simulink model "css"  (R2016a)
settings: Solver=ode45  StartTime=0.0  StopTime=inf  RelTol=1e-3
libraries: commfilt2 x3, commrflib2 x2, commrandsrc2 x2, commchan3 x1, commdigbbndam3 x1, dspspect3 x1
settings Model: Creator=NhatPham  LastModifiedBy=Nhat Pham
settings DataIOCC: LimitDataPoints=on  SaveFormat=Array
settings DebuggingCC: SolverPrmCheckMsg=warning
settings HardwareCC: ProdBitPerPointer=32  ProdLargestAtomicFloat=None  ProdIntDivRoundTo=Undefined  ProdEndianess=Unspecified  ProdWordSize=32  ProdHWDeviceType=32-bit Generic
settings ModelReferenceCC: PropagateSignalLabelsOutOfModel=off
settings ConfigComp: CovModelRefEnable=Off  CovSFcnEnable=off

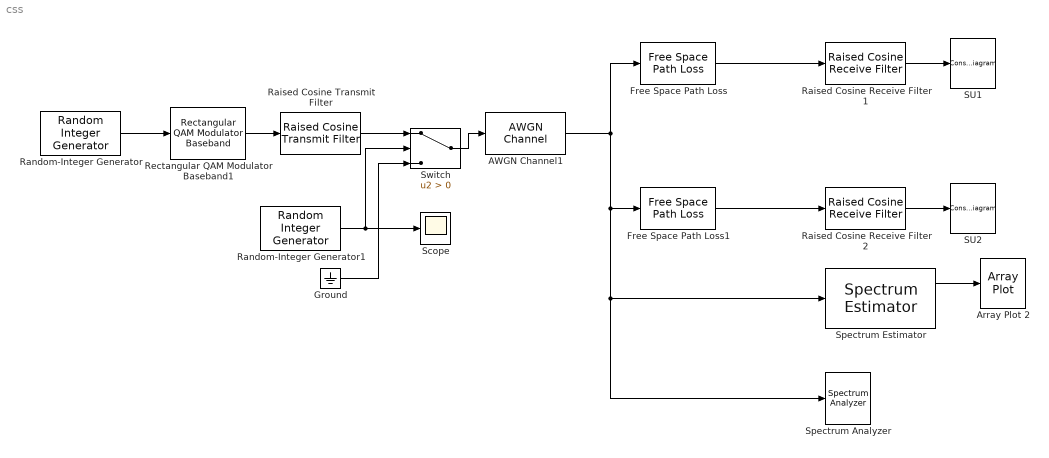
== system css ==
  AWGN Channel1 : commchan3/AWGN Channel  InputProcessing=Columns as channels (frame based)  seed=54321  noiseMode="Signal to noise ratio  (SNR)"  EbNodB=10  EsNodB=15  SNRdB=50  bitsPerSym=1  Ps=5  Tsym=.001  variance=1
  Array Plot 2 : ArrayPlot
  Free Space Path Loss : commrflib2/Free Space Path Loss  mode=Distance and Frequency  dB=10  d=50/1000  fc=2400
  Free Space Path Loss1 : commrflib2/Free Space Path Loss  mode=Distance and Frequency  dB=10  d=0.100  fc=2400
  Ground : Ground
  Raised Cosine Receive Filter 1 : commfilt2/Raised Cosine Receive Filter  filtType=Square root  R=0.2  filtSpan=10  N=8  downFactor=8  downOffset=0  filterGain=1  InputProcessing=Columns as channels (frame based)  RateOptions=Enforce single-rate processing  framing=Mute  checkCoeff=off  variableName=rcRxFilt  currentFiltSpan=10  D=5  inputOffset=0  sampMode=Mute  saveAsFlag=0  rateMode=Downsampling  checkGain=Normalized  launchFVT=on  roundingMode=Floor  overflowMode=off  coeffDataTypeStr=Inherit: Same word length as input  coeffMin=[]  coeffMax=[]  coeffLastDataTypeStr=Inherit: Same word length as input  accumDataTypeStr=Inherit: Same as product output  accumLastDataTypeStr=Inherit: Same as product output  outputDataTypeStr=Inherit: Same as accumulator  outputMin=[]  outputMax=[]  outputLastDataTypeStr=Inherit: Same as accumulator
  Raised Cosine Receive Filter 2 : commfilt2/Raised Cosine Receive Filter  filtType=Square root  R=0.2  filtSpan=10  N=8  downFactor=8  downOffset=0  filterGain=1  InputProcessing=Columns as channels (frame based)  RateOptions=Enforce single-rate processing  framing=Mute  checkCoeff=off  variableName=rcRxFilt1  currentFiltSpan=10  D=5  inputOffset=0  sampMode=Mute  saveAsFlag=0  rateMode=Downsampling  checkGain=Normalized  launchFVT=on  roundingMode=Floor  overflowMode=off  coeffDataTypeStr=Inherit: Same word length as input  coeffMin=[]  coeffMax=[]  coeffLastDataTypeStr=Inherit: Same word length as input  accumDataTypeStr=Inherit: Same as product output  accumLastDataTypeStr=Inherit: Same as product output  outputDataTypeStr=Inherit: Same as accumulator  outputMin=[]  outputMax=[]  outputLastDataTypeStr=Inherit: Same as accumulator
  Raised Cosine Transmit Filter : commfilt2/Raised Cosine Transmit Filter  filtType=Square root  R=0.2  filtSpan=10  N=8  filterGain=1  InputProcessing=Columns as channels (frame based)  RateOptions=Enforce single-rate processing  framing=Mute  checkCoeff=off  variableName=rcTxFilt  checkGain=Normalized  sampMode=Mute  saveAsFlag=0  currentFiltSpan=10  D=(10)/2  launchFVT=on  roundingMode=Floor  overflowMode=off  coeffDataTypeStr=Inherit: Same word length as input  coeffMin=[]  coeffMax=[]  coeffLastDataTypeStr=Inherit: Same word length as input  outputDataTypeStr=Inherit: Same as accumulator  outputMin=[]  outputMax=[]  outputLastDataTypeStr=Inherit: Same as accumulator
  Random-Integer Generator : commrandsrc2/Random Integer Generator  mul=16  seed=12345  Ts=1/500  frameBased=on  sampPerFrame=500  orient=off  outDataType=uint8
  Random-Integer Generator1 : commrandsrc2/Random Integer Generator  mul=2  seed=111  Ts=5  frameBased=off  sampPerFrame=1  orient=off  outDataType=boolean
  Rectangular QAM Modulator Baseband1 : commdigbbndam3/Rectangular QAM Modulator Baseband  M=16  InType=Integer  Enc=Binary  Mapping=[0:15]  PowType=Average Power  MinDist=2  AvgPow=1  PeakPow=1  Ph=0  outDtype=double  outWordLen=16  outUDDataType=sfix(16)  outFracLenMode=Best precision  outFracLen=15  outDataTypeStr=double  outLastDataTypeStr=double
  SU1 : ConstellationDiagram  Tag=ScatterPlot
  SU2 : ConstellationDiagram  Tag=ScatterPlot
  Scope : Scope
  Spectrum Analyzer : SpectrumAnalyzer
  Spectrum Estimator : dspspect3/Spectrum Estimator  SpectrumType=Power density  FrequencyResolutionMethod=Window length  RBW=5  WindowMode=Specify on dialog  WindowLength=1024  FFTLengthSource=Auto  FFTLength=1024  InheritSampleRate=on  SampleRate=44100  Window=Hann  SidelobeAttenuation=60  SpectralAverages=1  Overlap=0  ReferenceLoad=1  FrequencyRange=Centered  PowerUnits=dBm  OutputMaxHoldSpectrum=off  OutputMinHoldSpectrum=off  OutputFrequencyVector=on  OutputRBW=off  SimulateUsing=Interpreted execution
  Switch : Switch  Criteria=u2 > Threshold
  wires:
  Ground/1 -> Switch/3
  Random-Integer Generator1/1 -> Scope/1, Switch/2
  Rectangular QAM Modulator Baseband1/1 -> Raised Cosine Transmit Filter/1
  Random-Integer Generator/1 -> Rectangular QAM Modulator Baseband1/1
  Raised Cosine Receive Filter 1/1 -> SU1/1
  Raised Cosine Transmit Filter/1 -> Switch/1
  Switch/1 -> AWGN Channel1/1
  Free Space Path Loss/1 -> Raised Cosine Receive Filter 1/1
  Free Space Path Loss1/1 -> Raised Cosine Receive Filter 2/1
  Raised Cosine Receive Filter 2/1 -> SU2/1
  Spectrum Estimator/1 -> Array Plot 2/1
  AWGN Channel1/1 -> Spectrum Analyzer/1, Spectrum Estimator/1, Free Space Path Loss1/1, Free Space Path Loss/1
